simulink model "gm_opv_receiver_HDL_coder_input"  (R2023a)
settings: Solver=VariableStepDiscrete  StartTime=0.0  StopTime=10*(samples_per_frame/sample_rate)  RelTol=1e-3
undefined symbols (not defined in the file or in its folder): sample_rate
libraries: commrandsrc3 x2
settings Model: Creator=matt  LastModifiedBy=matt
settings OptimizationCC: BlockReduction=off  ConditionallyExecuteInputs=off  DefaultParameterBehavior=Inlined
settings DebuggingCC: AlgebraicLoopMsg=error  InheritedTsInSrcMsg=none
settings HardwareCC: ProdBitPerPointer=32  ProdBitPerSizeT=32  ProdBitPerPtrDiffT=32  ProdLargestAtomicFloat=None  ProdIntDivRoundTo=Undefined  ProdEndianess=Unspecified  ProdWordSize=32  ProdHWDeviceType=ASIC/FPGA->ASIC/FPGA  TargetBitPerLong=64  TargetBitPerPointer=64  TargetBitPerSizeT=64  TargetBitPerPtrDiffT=64  TargetLongLongMode=on  TargetIntDivRoundTo=Zero  TargetEndianess=LittleEndian  TargetWordSize=64  TargetHWDeviceType=Custom Processor->MATLAB Host Computer  ProdEqTarget=off

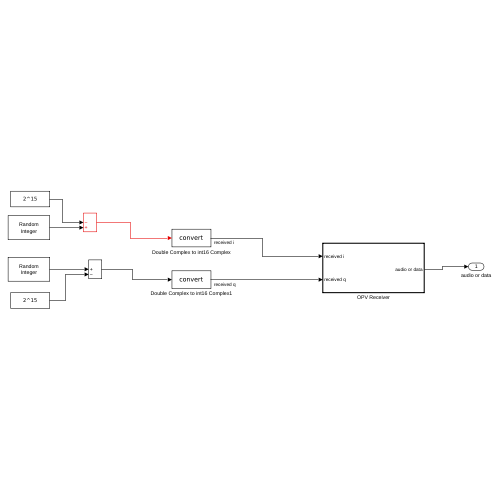
[thumbnail: Simulink's stored preview of the top-level diagram]
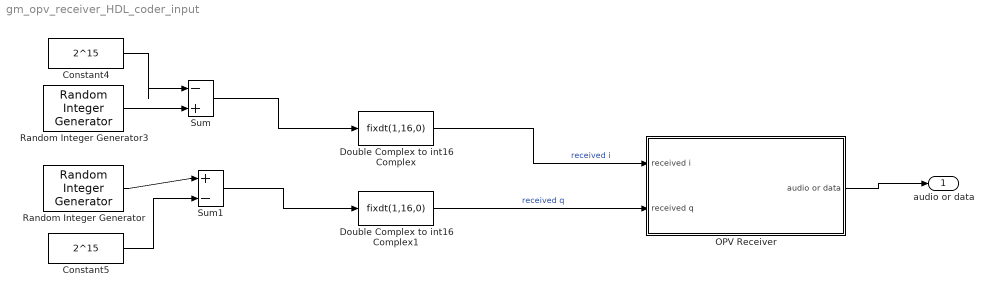
== system gm_opv_receiver_HDL_coder_input ==
  Constant4 : Constant  Value=2^15  SampleTime=1/sample_rate
  Constant5 : Constant  Value=2^15  SampleTime=1/sample_rate
  Double Complex to int16 Complex : DataTypeConversion  OutMin=[-32768]  OutMax=[32767]  OutDataTypeStr=fixdt(1,16,0)  RndMeth=Floor
  Double Complex to int16 Complex1 : DataTypeConversion  OutMin=[-32768]  OutMax=[32767]  OutDataTypeStr=fixdt(1,16,0)  RndMeth=Floor
  OPV Receiver : Subsystem  TreatAsAtomicUnit=on
      settings: LibrarySourceBlock=|
      | hdlsllib/Ports &
      | Subsystems/Subsystem
  Random Integer Generator : commrandsrc3/Random Integer Generator  SetSize=2^16  SeedSource=Auto  Seed=0  SampleTime=1/sample_rate  SamplesPerFrame=1  OutputDataType=double  SimulateUsing=Interpreted execution
  Random Integer Generator3 : commrandsrc3/Random Integer Generator  SetSize=2^16  SeedSource=Auto  Seed=0  SampleTime=1/sample_rate  SamplesPerFrame=1  OutputDataType=double  SimulateUsing=Interpreted execution
  Sum : Sum  Inputs=|-+
  Sum1 : Sum  Inputs=|+-
  audio or data : Outport
  wires:
  Double Complex to int16 Complex1/1 -> OPV Receiver/2(received q)  "received q"
  Double Complex to int16 Complex/1 -> OPV Receiver/1(received i)  "received i"
  OPV Receiver/1(audio or data) -> audio or data/1
  Constant5/1 -> Sum1/2
  Sum/1 -> Double Complex to int16 Complex/1
  Sum1/1 -> Double Complex to int16 Complex1/1
  Constant4/1 -> Sum/1
  Random Integer Generator/1 -> Sum1/1
  Random Integer Generator3/1 -> Sum/2

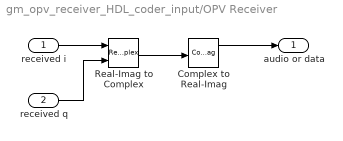
== system gm_opv_receiver_HDL_coder_input/OPV Receiver ==
  received i : Inport
  received q : Inport  Port=2
  Complex to Real-Imag : ComplexToRealImag
  Real-Imag to Complex : RealImagToComplex
  audio or data : Outport
  wires:
  Complex to Real-Imag/1 -> audio or data/1
  Real-Imag to Complex/1 -> Complex to Real-Imag/1
  received q/1 -> Real-Imag to Complex/2
  received i/1 -> Real-Imag to Complex/1
